simulink model "AOOR_testing"  (R2022a)
settings: Solver=FixedStepAuto  StartTime=0.0  StopTime=10.0  FixedStep=1e-3  RelTol=1e-3  EnableMultiTasking=on
undefined symbols (not defined in the file): D10, D11, D2, D4, D5, D8, D9, PTA0, PTA2, PTB23, PTB9, PTC4, PTD0, PTD2
libraries: frdmk64flib x7
settings Model: ExtModeTrigDuration=5  Creator=kemij  LastModifiedBy=bmile
settings OptimizationCC: EnhancedBackFolding=on  PassReuseOutputArgsAs=Individual arguments  ZeroExternalMemoryAtStartup=off  ZeroInternalMemoryAtStartup=off  MaxStackSize=64  OptimizeBlockOrder=speed  DifferentSizesBufferReuse=on  OptimizationCustomize=off  EfficientTunableParamExpr=on
settings DebuggingCC: ParameterTunabilityLossMsg=error
settings HardwareCC: ProdBitPerPointer=32  ProdBitPerSizeT=32  ProdBitPerPtrDiffT=32  ProdLargestAtomicInteger=Long  ProdLargestAtomicFloat=Double  ProdWordSize=32  ProdHWDeviceType=ARM Compatible->ARM Cortex
settings SFSimCC: MATLABDynamicMemAlloc=off
settings RTWCC: SystemTargetFile=ert.tlc  HardwareBoard=NXP FRDM-K64F  TLCOptions="-aInlineSetEventsForThisBaseRateFcn=TLC_FALSE -aSuppressMultiTaskScheduler=TLC_FALSE  -aRateBasedStepFcn=0"  TemplateMakefile=ert_default_tmf  Toolchain=GNU Tools for ARM Embedded Processors
settings CodeAppCC: ForceParamTrailComments=on  IgnoreCustomStorageClasses=off  OperatorAnnotations=on  SimulinkDataObjDesc=on  SFDataObjDesc=on  InsertBlockDesc=on
settings ERTTargetCC: ExtModeTransport=4  ExtModeMexFile=sendToCommService

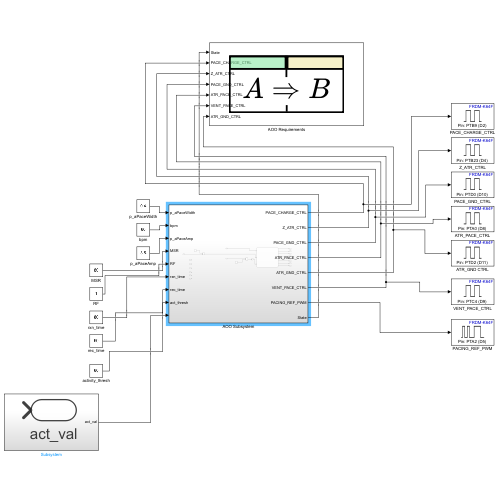
[thumbnail: Simulink's stored preview of the top-level diagram]
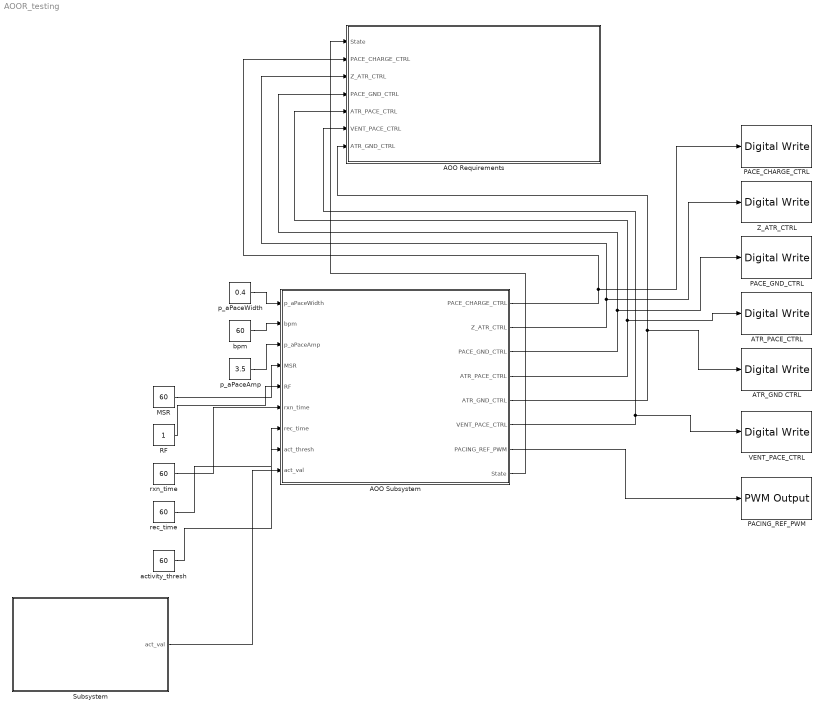
== system AOOR_testing ==
  AOO Requirements : Requirements Table  TreatAsAtomicUnit=on
  AOO Subsystem : Subsystem
  ATR_GND CTRL : frdmk64flib/Digital Write  Whichpin=PTD2 (D11)
  ATR_PACE_CTRL : frdmk64flib/Digital Write  Whichpin=PTA0 (D8)
  MSR : Constant  Value=60
  PACE_CHARGE_CTRL : frdmk64flib/Digital Write  Whichpin=PTB9 (D2)
  PACE_GND_CTRL : frdmk64flib/Digital Write  Whichpin=PTD0 (D10)
  PACING_REF_PWM : frdmk64flib/PWM Output  Whichpin=PTA2 (D5)  InitialFrequency=2000  InitialDutyCycle=0
  RF : Constant
  Subsystem : Subsystem
  VENT_PACE_CTRL : frdmk64flib/Digital Write  Whichpin=PTC4 (D9)
  Z_ATR_CTRL : frdmk64flib/Digital Write  Whichpin=PTB23 (D4)
  activity_thresh : Constant  Value=60
  bpm : Constant  Value=60
  p_aPaceAmp : Constant  Value=3.5
  p_aPaceWidth : Constant  Value=0.4
  rec_time : Constant  Value=60
  rxn_time : Constant  Value=60
  wires:
  p_aPaceAmp/1 -> AOO Subsystem/3(p_aPaceAmp)
  AOO Subsystem/5(ATR_GND_CTRL) -> AOO Requirements/7(ATR_GND_CTRL), ATR_GND CTRL/1
  AOO Subsystem/4(ATR_PACE_CTRL) -> AOO Requirements/5(ATR_PACE_CTRL), ATR_PACE_CTRL/1
  AOO Subsystem/3(PACE_GND_CTRL) -> AOO Requirements/4(PACE_GND_CTRL), PACE_GND_CTRL/1
  AOO Subsystem/2(Z_ATR_CTRL) -> AOO Requirements/3(Z_ATR_CTRL), Z_ATR_CTRL/1
  AOO Subsystem/1(PACE_CHARGE_CTRL) -> AOO Requirements/2(PACE_CHARGE_CTRL), PACE_CHARGE_CTRL/1
  p_aPaceWidth/1 -> AOO Subsystem/1(p_aPaceWidth)
  bpm/1 -> AOO Subsystem/2(bpm)
  AOO Subsystem/6(VENT_PACE_CTRL) -> AOO Requirements/6(VENT_PACE_CTRL), VENT_PACE_CTRL/1
  AOO Subsystem/7(PACING_REF_PWM) -> PACING_REF_PWM/1
  AOO Subsystem/8(State) -> AOO Requirements/1(State)
  MSR/1 -> AOO Subsystem/4(MSR)
  RF/1 -> AOO Subsystem/5(RF)
  rxn_time/1 -> AOO Subsystem/6(rxn_time)
  rec_time/1 -> AOO Subsystem/7(rec_time)
  activity_thresh/1 -> AOO Subsystem/8(act_thresh)
  Subsystem/1(act_val) -> AOO Subsystem/9(act_val)

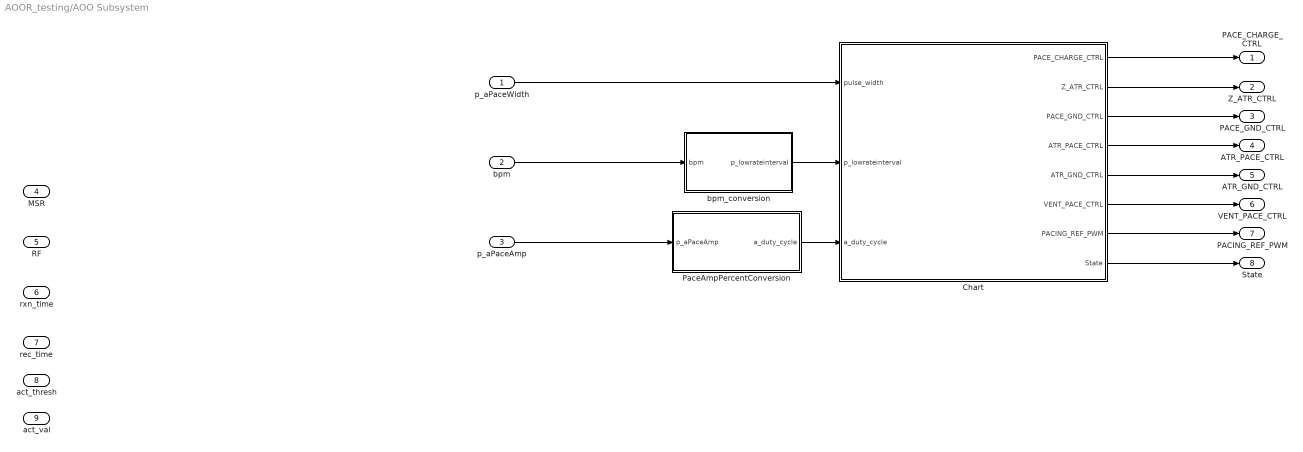
== system AOOR_testing/AOO Subsystem ==
  p_aPaceWidth : Inport
  bpm : Inport  Port=2
  p_aPaceAmp : Inport  Port=3
  MSR : Inport  Port=4
  RF : Inport  Port=5
  rxn_time : Inport  Port=6
  rec_time : Inport  Port=7
  act_thresh : Inport  Port=8
  act_val : Inport  Port=9
  Chart : Stateflow chart  TreatAsAtomicUnit=on
      settings: PortSchema="{\"entries\":[{\"content\":{\"sides\":[{\"content\":{\"connectorIds\":[\"In1\",\"In3\",\"In2\"]},\"type\":\"ConnectorPlacement.EquallySpacedRectSide\",\"uuid\":\"7e75a948-41f4-4c79-9882-3d88287f3c70\"},{\"content\":{\"connectorIds\":[\"Out1\",\"Out2\",\"Out3\",\"Out4\",\"Out5\",\"Out6\",\"Out8\",\"Out7\"],\"side\":\"RIGHT\"},\"type\":\"ConnectorPlacement.EquallySpacedRectSide\",\"uuid\":\"511746b0-37fa-476a-b800-6cf6e50abaf9\"},{\"content\":{\"connectorIds\":[],\"side\":\"TOP\"},\"type\":\"ConnectorPlacement.EquallySpacedRectSide\",\"uuid\":\"11666b54-d2f4-4011-ac63-76655f465a3e\"}]},\"type\":\"ConnectorPlacement.EquallySpacedConnector\",\"uuid\":\"d0a37cb0-b7e8-4d7b-82f4-74da072fb485\"}],\"packageUris\":[\"http://schema.mathworks.com/mf0/Connector/R2020b\"],\"version\":\"1.0\"}"
  PaceAmpPercentConversion : Subsystem
  bpm_conversion : Subsystem
  PACE_CHARGE_CTRL : Outport
  Z_ATR_CTRL : Outport  Port=2
  PACE_GND_CTRL : Outport  Port=3
  ATR_PACE_CTRL : Outport  Port=4
  ATR_GND_CTRL : Outport  Port=5
  VENT_PACE_CTRL : Outport  Port=6
  PACING_REF_PWM : Outport  Port=7
  State : Outport  Port=8
  wires:
  p_aPaceWidth/1 -> Chart/1(pulse_width)
  Chart/1(PACE_CHARGE_CTRL) -> PACE_CHARGE_CTRL/1
  Chart/2(Z_ATR_CTRL) -> Z_ATR_CTRL/1
  Chart/3(PACE_GND_CTRL) -> PACE_GND_CTRL/1
  Chart/4(ATR_PACE_CTRL) -> ATR_PACE_CTRL/1
  Chart/5(ATR_GND_CTRL) -> ATR_GND_CTRL/1
  Chart/6(VENT_PACE_CTRL) -> VENT_PACE_CTRL/1
  Chart/8(PACING_REF_PWM) -> PACING_REF_PWM/1
  Chart/7(State) -> State/1
  PaceAmpPercentConversion/1(a_duty_cycle) -> Chart/2(a_duty_cycle)
  p_aPaceAmp/1 -> PaceAmpPercentConversion/1(p_aPaceAmp)
  bpm/1 -> bpm_conversion/1(bpm)
  bpm_conversion/1(p_lowrateinterval) -> Chart/3(p_lowrateinterval)

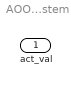
== system AOOR_testing/Subsystem ==
  act_val : Outport

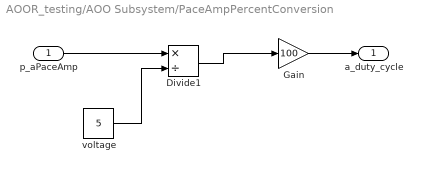
== system AOOR_testing/AOO Subsystem/PaceAmpPercentConversion ==
  p_aPaceAmp : Inport
  Divide1 : Product  Inputs=*/
  Gain : Gain  Gain=100
  voltage : Constant  Value=5
  a_duty_cycle : Outport
  wires:
  voltage/1 -> Divide1/2
  Divide1/1 -> Gain/1
  p_aPaceAmp/1 -> Divide1/1
  Gain/1 -> a_duty_cycle/1

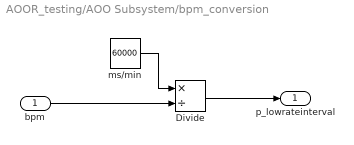
== system AOOR_testing/AOO Subsystem/bpm_conversion ==
  bpm : Inport
  Divide : Product  Inputs=*/
  ms/min : Constant  Value=60000
  p_lowrateinterval : Outport
  wires:
  ms/min/1 -> Divide/1
  bpm/1 -> Divide/2
  Divide/1 -> p_lowrateinterval/1

== stateflow chart AOOR_testing/AOO Requirements ==
  (default) -> (junction 1073743090)
  (junction 1073743090) -> (junction 1073743091) : {
      | % SF_REQ_REV_07
      | }
  (junction 1073743091) -> (junction 1073743093) : {
      | % HEADER_ASSIGNMENTS
      |
      | }
  (junction 1073743093) -> (junction 1073743095) : {
      | % START_A_4
      | }
  (junction 1073743095) -> (junction 1073743097) : {
      | }
  (junction 1073743097) -> (junction 1073743099)
  (junction 1073743099) -> (junction 1073743101) : {
      | }
  (junction 1073743101) -> (junction 1073743103) : {
      | % END_A_4
      | }
  (junction 1073743103) -> (junction 1073743206) : {
      | % START_R_1
      | }
  (junction 1073743206) -> (junction 1073743208) : {
      | }
  (junction 1073743208) -> (junction 1073743210)
  (junction 1073743210) -> (junction 1073743212) [order 1] : [(((State) == (0)))]
  (junction 1073743210) -> (junction 1073743218) [order 2]
  (junction 1073743212) -> (junction 1073743214) : {
      | reqtable_postcondition((((ATR_PACE_CTRL) == (false))) && (((VENT_PACE_CTRL) == (false))) && (((PACE_CHARGE_CTRL) == (true))) && (((ATR_GND_CTRL) == (true))) && (((PACE_GND_CTRL) == (true))) && (((Z_ATR_CTRL) == (false))), 'R:1');
      |
      |
      | }
  (junction 1073743214) -> (junction 1073743216) : {
      | }
  (junction 1073743216) -> (junction 1073743218)
  (junction 1073743218) -> (junction 1073743220)
  (junction 1073743220) -> (junction 1073743222) : {
      | % END_R_1
      | }
  (junction 1073743222) -> (junction 1073743123) : {
      | % START_R_7
      | }
  (junction 1073743123) -> (junction 1073743125) : {
      | }
  (junction 1073743125) -> (junction 1073743127)
  (junction 1073743127) -> (junction 1073743129) [order 1] : [(((State) == (1)))]
  (junction 1073743127) -> (junction 1073743135) [order 2]
  (junction 1073743129) -> (junction 1073743131) : {
      | reqtable_postcondition((((ATR_PACE_CTRL) == (true))) && (((VENT_PACE_CTRL) == (false))) && (((PACE_CHARGE_CTRL) == (false))) && (((ATR_GND_CTRL) == (false))) && (((PACE_GND_CTRL) == (true))) && (((Z_ATR_CTRL) == (false))), 'R:2');
      |
      |
      | }
  (junction 1073743131) -> (junction 1073743133) : {
      | }
  (junction 1073743133) -> (junction 1073743135)
  (junction 1073743135) -> (junction 1073743137)
  (junction 1073743137) -> (junction 1073743139) : {
      | % END_R_7
      | }
  data: State input; PACE_CHARGE_CTRL input; Z_ATR_CTRL input; PACE_GND_CTRL input; ATR_PACE_CTRL input; VENT_PACE_CTRL input; ATR_GND_CTRL input

== stateflow chart AOOR_testing/AOO Subsystem/Chart ==
  state Charging_Discharging
    entry:
    ATR_PACE_CTRL = false
    VENT_PACE_CTRL=false
    PACE_CHARGE_CTRL = true
    ATR_GND_CTRL = true
    PACE_GND_CTRL = true
    Z_ATR_CTRL=false
    PACING_REF_PWM =a_duty_cycle
    State = 0
  state Pace_Heart
    entry:
    ATR_PACE_CTRL = true
    PACE_CHARGE_CTRL = false
    PACE_GND_CTRL = true
    ATR_GND_CTRL = false
    State = 1
  (default) -> Charging_Discharging
  Charging_Discharging -> Pace_Heart : after(p_lowrateinterval-pulse_width,msec)
  Pace_Heart -> Charging_Discharging : after(pulse_width,msec)
  data: pulse_width input; PACE_CHARGE_CTRL output boolean; Z_ATR_CTRL output boolean; PACE_GND_CTRL output boolean; ATR_PACE_CTRL output boolean; ATR_GND_CTRL output boolean; VENT_PACE_CTRL output; a_duty_cycle input; State output; p_lowrateinterval input; PACING_REF_PWM output
